simulink model "Electrical_System_2018b_obfs"  (R2019b)
settings: Solver=VariableStepAuto  StartTime=0.0  StopTime=5  RelTol=1e-3  AbsTol=1e-3  EnableMultiTasking=on
InitFcn:
  | Steady_State_Initialisation;
StopFcn:
  | %sscexplore(simlog);
  | %Logging
undefined symbols (not defined in the file): abrlhklxvp, aexgmhuedq, afmfmjnutg, afpphrjpnc, ahuxbyvruc, alarvljztt, amxnyqmnuw, aodrlwvqie, aolhmuplyq, aqpmguuqkg, auesgwirzl, aurophlnng, awamelrhru, ayfhvxflxn, azxkacuhqc, babszerikg, bawhdqanwq, bevoqecvei, bltjvqbchx, bmqsuewujl, bsmyqjfgnf, btvjbsmnve, bywgxqeadw, bziaduxaer, bzmcmdqocb, bzsvyvetat, ccsjnrbsih, cdvenygxwh, cedkrnslhx, cjheorclzs, cjrdshrtqx, ckhavyhcza, ckxewznhlz, cmrcgyiplk, conenicnws, cqkejbgjnn, csfnuwymhe, cunupkhwbh, cwzfvzuxxh, dcadmadufn, dcfponivnv, ddtrqjrhjn, dfhoxvkqas, dfrhtcwpne, dfvomcagjv, djijwylxea, dnmeqksrrm, dnzewbdkaa, dsqcykyxav, dtswwlttmm, ecumpidjtv, edegaywrct, ejjjsmnejc, eknqnehjdz, emvdetzouf, esxbqkbahr, etnkkbreiq, eunoiiiirw, ewewcuedir, fatkfxdhtc ... (+386)
libraries: fl_lib x802, ee_lib x362, fl_ps_legacy_lib x160, nesl_utility x85
(part 24 of 26)

== system Electrical_System_2018b_obfs/Redacted_1221/Redacted_7996/Redacted_9242/Redacted_38/Redacted_8107/Redacted_7529 ==
  Redacted_1084 : ee_lib/Semiconductors & Converters/Diode  ModelType=izdobyzqle  Vf=evihkhstbw V  Ron=vuuzcskhxp Ohm  Goff=mlnvudefzh S  prmExp=lejtfyvyux  I12=tabfzyvjjw A  V12=fmhjbmpmqb V  IS=owmyvxeefr A  ec=svhshwyrgx  I1=ljwwgiysfr A  V1=cxpndjgyrh V  RS=xmnymghsco Ohm  Tmeas=zghhcluqyd degC  N_series=cpqweisfkm  N_parallel=lexvmnvtgk  Rz=qmwaibykde Ohm  BV=drbkvafvno V  C_param=xxddurxsbn  CJ=xdxqdbopkt pF  CJ0=kptwwgjzso pF  VJ=hkmlapdavl V  Mgrad=vyzsmtybaj  Vvec=idvcnbeqxi V  Cvec=lhhotedrtn pF  FC=bewrjixdsy  Q_param=ivgezzsvid  iRM=kttgtaurdl A  iF=feyuhnjntw A  didt=wzaronjtgo A/us  trr_factor=xjeyfathbr  trr=gmgemqpikq ns  Qrr=psqfrowxwi s*uA  TT=klclxejlrf ns  tau=dytmmyuhbl ns  T_param=gahisfowsc  IS_T2=cvrsutiwlp A  I1_T2=lhcryknhzp A  V1_T2=nabkspnaxp V  Tmeas2=yxgzayqlzi degC  EG_param=qwryskkgkm  EG=oxgfzaipim eV  XTI_param=bjoagcqjsw  XTI=ycmlwmcwwf  dBVdT=dotvxllash V/K  Tdevice=ezkzuymnag degC  i_specify=off  i_priority=None  i=daydkonpxs A  i_nominal_specify=off  i_nominal_unit=A  i_nominal_value=blmtdukctw  v_specify=off  v_priority=None  v=akgpvqsdrg V  v_nominal_specify=off  v_nominal_unit=V  v_nominal_value=lygvltjuxz  i_capacitor_specify=off  i_capacitor_priority=None  i_capacitor=btazvuzoqw A  i_capacitor_nominal_specify=off  i_capacitor_nominal_unit=A  i_capacitor_nominal_value=mpfscvienm  v_capacitor_specify=off  v_capacitor_priority=None  v_capacitor=fmmkhztbpm V  v_capacitor_nominal_specify=off  v_capacitor_nominal_unit=V  v_capacitor_nominal_value=ltvznzjvwn  power_dissipated_specify=off  power_dissipated_priority=None  power_dissipated=jxwbertlfp W  power_dissipated_nominal_specify=off  power_dissipated_nominal_unit=W  power_dissipated_nominal_value=qtoemtvmie  thermal_network_parameterization=vtcsjudzim  Rth=heeowetwuv K/W  Rth_Foster=ruqyjqugrl K/W  thermal_mass_parameterization=envbmlquin  thermal_mass=kwknucpqzf J/K  thermal_mass_Foster=cqdqbkuljl J/K  thermal_time_constant=ngzwrugeai s  thermal_time_constant_Foster=bpqkuoqgpu s  thermal_mass_initial_temperatures=rhqgsoeffv degC
      settings: SourceProductName=Simscape Electrical  InternalSimscapePortConfiguration="{\"Bottom\":[],\"Left\":[{\"id\":\"p\",\"label\":\"\",\"type\":\"foundation.electrical.electrical\"},{\"id\":\"H\",\"label\":\"H\",\"type\":\"foundation.thermal.thermal\"}],\"Right\":[{\"id\":\"n\",\"label\":\"\",\"type\":\"foundation.electrical.electrical\"}],\"Top\":[]}"
  Redacted_1116 : ee_lib/Semiconductors & Converters/Diode  ModelType=fezxkqjgqt  Vf=fxigmtorpi V  Ron=gczbijkgdb Ohm  Goff=eezdenrgyt S  prmExp=mooftzwsze  I12=hrjfyjjrls A  V12=rpjtpkqqat V  IS=wddelpkxcd A  ec=wnwrwrhrqv  I1=lxjmeqhfps A  V1=hwunywjuky V  RS=qeymtoopbm Ohm  Tmeas=moiijwwbbr degC  N_series=tpmlovrlqd  N_parallel=mfzinvasat  Rz=ovydxazbex Ohm  BV=pxxjbuwfqz V  C_param=qpcursofjw  CJ=xcjuvsuivt pF  CJ0=izhwoolfnz pF  VJ=vpiestyydi V  Mgrad=cktkfzulrn  Vvec=sciesnzgxa V  Cvec=ffirljqncp pF  FC=ggluskildl  Q_param=ivvyfxrgkf  iRM=vqdtwwvmky A  iF=pvrysfcrbt A  didt=aeuywekxid A/us  trr_factor=nqhyqwmkdj  trr=iqctnvzxva ns  Qrr=isykhlqcxv s*uA  TT=ebdjbikpxl ns  tau=braofdeijp ns  T_param=rwhudzydrl  IS_T2=ahyaxsqykv A  I1_T2=yqxbhliehb A  V1_T2=cahaepnczu V  Tmeas2=rcpxcpgkrc degC  EG_param=ajpcsxcgmn  EG=mkbrzouimp eV  XTI_param=fgrnhizmgq  XTI=rtivxbansn  dBVdT=bztvayfwko V/K  Tdevice=fwkbokttbz degC  i_specify=off  i_priority=None  i=frjerhxssh A  i_nominal_specify=off  i_nominal_unit=A  i_nominal_value=xtkoagasgf  v_specify=off  v_priority=None  v=ltequmallb V  v_nominal_specify=off  v_nominal_unit=V  v_nominal_value=nmmakwdacx  i_capacitor_specify=off  i_capacitor_priority=None  i_capacitor=oexcyamlgf A  i_capacitor_nominal_specify=off  i_capacitor_nominal_unit=A  i_capacitor_nominal_value=tsglkvwluo  v_capacitor_specify=off  v_capacitor_priority=None  v_capacitor=uttypvaate V  v_capacitor_nominal_specify=off  v_capacitor_nominal_unit=V  v_capacitor_nominal_value=rmuymllcxy  power_dissipated_specify=off  power_dissipated_priority=None  power_dissipated=pikztcggua W  power_dissipated_nominal_specify=off  power_dissipated_nominal_unit=W  power_dissipated_nominal_value=wdovbxesnv  thermal_network_parameterization=jzuiubyezr  Rth=zuswrtrzus K/W  Rth_Foster=mncqifigaw K/W  thermal_mass_parameterization=xdyzfyucfr  thermal_mass=digaqnegbt J/K  thermal_mass_Foster=rlibwejjxp J/K  thermal_time_constant=dtpvzfxfdr s  thermal_time_constant_Foster=lltkuepcfr s  thermal_mass_initial_temperatures=qrjsznixcz degC
      settings: SourceProductName=Simscape Electrical  InternalSimscapePortConfiguration="{\"Bottom\":[],\"Left\":[{\"id\":\"p\",\"label\":\"\",\"type\":\"foundation.electrical.electrical\"},{\"id\":\"H\",\"label\":\"H\",\"type\":\"foundation.thermal.thermal\"}],\"Right\":[{\"id\":\"n\",\"label\":\"\",\"type\":\"foundation.electrical.electrical\"}],\"Top\":[]}"
  Redacted_3535 : ee_lib/Passive/Thermal/Thermal Resistor  R=nnovauibfc K/W  T_specify=off  T_priority=None  T=smooypmoft K  T_nominal_specify=off  T_nominal_unit=K  T_nominal_value=kuntnrwjbm  Q_specify=off  Q_priority=None  Q=ffwudhgepl W  Q_nominal_specify=off  Q_nominal_unit=W  Q_nominal_value=dtpumxdoon
      settings: SourceProductName=Simscape Electrical  SourceProductBaseCode=PS  InternalSimscapePortConfiguration="{\"Bottom\":[],\"Left\":[{\"id\":\"A\",\"label\":\"A\",\"type\":\"foundation.thermal.thermal\"}],\"Right\":[{\"id\":\"B\",\"label\":\"B\",\"type\":\"foundation.thermal.thermal\"}],\"Top\":[]}"
  Redacted_4646 : fl_lib/Electrical/Electrical Elements/Switch  R_closed=pqgaemrczs Ohm  G_open=ijstyudrez 1/Ohm  Threshold=xtptocpmir  i_specify=off  i_priority=None  i=ciwbetxiqp A  i_nominal_specify=off  i_nominal_unit=A  i_nominal_value=enaqgcdnlz  v_specify=off  v_priority=None  v=vzxbmtbrih V  v_nominal_specify=off  v_nominal_unit=V  v_nominal_value=wsynujvvrc
      settings: SourceProductName=Simscape
  Redacted_5773 : ee_lib/Passive/Thermal/Thermal Resistor  R=edegaywrct K/W  T_specify=off  T_priority=None  T=ckxewznhlz K  T_nominal_specify=off  T_nominal_unit=K  T_nominal_value=gkohcrexhh  Q_specify=off  Q_priority=None  Q=ubkoftignu W  Q_nominal_specify=off  Q_nominal_unit=W  Q_nominal_value=dmlagltzis
      settings: SourceProductName=Simscape Electrical  SourceProductBaseCode=PS  InternalSimscapePortConfiguration="{\"Bottom\":[],\"Left\":[{\"id\":\"A\",\"label\":\"A\",\"type\":\"foundation.thermal.thermal\"}],\"Right\":[{\"id\":\"B\",\"label\":\"B\",\"type\":\"foundation.thermal.thermal\"}],\"Top\":[]}"
  Redacted_6378 : fl_lib/Electrical/Electrical Elements/Switch  R_closed=whblxebmyo Ohm  G_open=pswlapjyse 1/Ohm  Threshold=pwweavvhgn  i_specify=off  i_priority=None  i=elbzoqtfyk A  i_nominal_specify=off  i_nominal_unit=A  i_nominal_value=sbenumnblt  v_specify=off  v_priority=None  v=vclonruutc V  v_nominal_specify=off  v_nominal_unit=V  v_nominal_value=xzmfluzccj
      settings: SourceProductName=Simscape
  Redacted_6493 : ee_lib/Semiconductors & Converters/Diode  ModelType=vttiaricbl  Vf=ogmshccous V  Ron=clhmvbtmpj Ohm  Goff=qlartobjid S  prmExp=yehkiyfwrf  I12=uxupgfdefd A  V12=fnuyckqxoq V  IS=gijoawrwfl A  ec=jacbxiiccp  I1=fgncvolvfb A  V1=onmmvewocq V  RS=otizmpmqay Ohm  Tmeas=kapmscogpw degC  N_series=qithjwaybs  N_parallel=gzsiinkylg  Rz=mycurxzcbk Ohm  BV=rewmblcdnc V  C_param=whbhsgwygj  CJ=vcfjucyupa pF  CJ0=xlhglqasyv pF  VJ=qosroxbxnj V  Mgrad=hkxiwvlmct  Vvec=oruqsfqddv V  Cvec=sashthzyhc pF  FC=xhlcguewdu  Q_param=ixrezpchhb  iRM=djiqriviqu A  iF=hegkfqrgrh A  didt=xbnqhutjlk A/us  trr_factor=dzlursyiar  trr=ecuaptzqel ns  Qrr=imqebfbhyx s*uA  TT=dymphevecl ns  tau=sblfgxlvjk ns  T_param=xyqfplnupv  IS_T2=uxlhlnzgja A  I1_T2=cyfpvxxmef A  V1_T2=dbwddhswgd V  Tmeas2=zlvkqtpnfx degC  EG_param=fcgsavfugx  EG=jbtqkskxko eV  XTI_param=buvkrschfc  XTI=qctkrmjsmi  dBVdT=kyilrmqoag V/K  Tdevice=tvzbjueohw degC  i_specify=off  i_priority=None  i=wgxzavfjwv A  i_nominal_specify=off  i_nominal_unit=A  i_nominal_value=zeyksugkif  v_specify=off  v_priority=None  v=knzxvrfofm V  v_nominal_specify=off  v_nominal_unit=V  v_nominal_value=chjlmmweiu  i_capacitor_specify=off  i_capacitor_priority=None  i_capacitor=mednscufnd A  i_capacitor_nominal_specify=off  i_capacitor_nominal_unit=A  i_capacitor_nominal_value=leufklsnbm  v_capacitor_specify=off  v_capacitor_priority=None  v_capacitor=xrcvmsmjec V  v_capacitor_nominal_specify=off  v_capacitor_nominal_unit=V  v_capacitor_nominal_value=tbidastozp  power_dissipated_specify=off  power_dissipated_priority=None  power_dissipated=hpegcrwzwe W  power_dissipated_nominal_specify=off  power_dissipated_nominal_unit=W  power_dissipated_nominal_value=ueblnqxpvf  thermal_network_parameterization=hkgyvucefr  Rth=bprjyiudmm K/W  Rth_Foster=bqwxkgbgel K/W  thermal_mass_parameterization=gnzfaualyz  thermal_mass=qgoqgvzmhv J/K  thermal_mass_Foster=lrajjjlskm J/K  thermal_time_constant=ffhhmbgnyr s  thermal_time_constant_Foster=dwjhaccnar s  thermal_mass_initial_temperatures=clzednejpb degC
      settings: SourceProductName=Simscape Electrical  InternalSimscapePortConfiguration="{\"Bottom\":[],\"Left\":[{\"id\":\"p\",\"label\":\"\",\"type\":\"foundation.electrical.electrical\"},{\"id\":\"H\",\"label\":\"H\",\"type\":\"foundation.thermal.thermal\"}],\"Right\":[{\"id\":\"n\",\"label\":\"\",\"type\":\"foundation.electrical.electrical\"}],\"Top\":[]}"
  Redacted_6995 : ee_lib/Semiconductors & Converters/Diode  ModelType=jutammamgf  Vf=phixztrybu V  Ron=wnueokvcjp Ohm  Goff=tlbagzjnli S  prmExp=qepetuupwd  I12=pipfumlpkp A  V12=cvdomcruuy V  IS=caphgfqgul A  ec=bfsyyglqre  I1=chsqwrduxs A  V1=pnvjrtaaxm V  RS=lnonjcbaes Ohm  Tmeas=uqgbdgyiqe degC  N_series=wzcnpegdoc  N_parallel=vzpnmjfana  Rz=jvagvrqcvr Ohm  BV=iowbeuhkbn V  C_param=zuyiiufywv  CJ=iafdabsqml pF  CJ0=krrwskzkzk pF  VJ=hcozynotnd V  Mgrad=qgebppotct  Vvec=rsjrazbslf V  Cvec=tqthplanse pF  FC=ggxesrxcvy  Q_param=npdtukbqqy  iRM=baufngyjqn A  iF=eaqdcbooap A  didt=zpmwgjwvhg A/us  trr_factor=lxzhpepuka  trr=lxionuhlzp ns  Qrr=cedutijpwi s*uA  TT=unwcmeqxzu ns  tau=bqcttgeatr ns  T_param=hnuznnjugk  IS_T2=heqzetlzuz A  I1_T2=zuzqagssvf A  V1_T2=jebzqvibaa V  Tmeas2=liqnbtkzkz degC  EG_param=paovebrsxo  EG=afafawlgir eV  XTI_param=eznhhwiwyq  XTI=pnvwrinkhd  dBVdT=ncvzhuvhdd V/K  Tdevice=xjszywknrp degC  i_specify=off  i_priority=None  i=ksmvescqii A  i_nominal_specify=off  i_nominal_unit=A  i_nominal_value=vdbtoezmns  v_specify=off  v_priority=None  v=mjrlqidlhj V  v_nominal_specify=off  v_nominal_unit=V  v_nominal_value=kpyhvjeelx  i_capacitor_specify=off  i_capacitor_priority=None  i_capacitor=rleowstiyj A  i_capacitor_nominal_specify=off  i_capacitor_nominal_unit=A  i_capacitor_nominal_value=cqjcqxpbep  v_capacitor_specify=off  v_capacitor_priority=None  v_capacitor=atjaslazmh V  v_capacitor_nominal_specify=off  v_capacitor_nominal_unit=V  v_capacitor_nominal_value=wpxewlzklj  power_dissipated_specify=off  power_dissipated_priority=None  power_dissipated=mwdylpnyws W  power_dissipated_nominal_specify=off  power_dissipated_nominal_unit=W  power_dissipated_nominal_value=jrnlbozeni  thermal_network_parameterization=dbphpnpgiy  Rth=xxmcnnlxls K/W  Rth_Foster=owybowsyqi K/W  thermal_mass_parameterization=fipqtfbsom  thermal_mass=sufocoiqer J/K  thermal_mass_Foster=kpdllifdhl J/K  thermal_time_constant=miladgbser s  thermal_time_constant_Foster=ttjplmfpfh s  thermal_mass_initial_temperatures=yzetsrudhm degC
      settings: SourceProductName=Simscape Electrical  InternalSimscapePortConfiguration="{\"Bottom\":[],\"Left\":[{\"id\":\"p\",\"label\":\"\",\"type\":\"foundation.electrical.electrical\"},{\"id\":\"H\",\"label\":\"H\",\"type\":\"foundation.thermal.thermal\"}],\"Right\":[{\"id\":\"n\",\"label\":\"\",\"type\":\"foundation.electrical.electrical\"}],\"Top\":[]}"
  Redacted_7501 : fl_lib/Electrical/Electrical Elements/Switch  R_closed=hkpufaysry Ohm  G_open=gpzouyuqvs 1/Ohm  Threshold=qzaeawbkdg  i_specify=off  i_priority=None  i=gtsknxhqqy A  i_nominal_specify=off  i_nominal_unit=A  i_nominal_value=zlbtgeochj  v_specify=off  v_priority=None  v=dywgqxyfrf V  v_nominal_specify=off  v_nominal_unit=V  v_nominal_value=tmhxabklck
      settings: SourceProductName=Simscape
  Redacted_7912 : ee_lib/Semiconductors & Converters/Diode  ModelType=rwagzwdqyn  Vf=iprlzxekyz V  Ron=ezbutranua Ohm  Goff=dhqmfjsjtj S  prmExp=cuexlqtxbd  I12=huvborskst A  V12=yjowgrbbok V  IS=recqqdaika A  ec=maqoiaeowd  I1=dfgsziufhg A  V1=jfgkxmlxal V  RS=rwxzegglbh Ohm  Tmeas=jioffbrnci degC  N_series=fvxphqozbm  N_parallel=klvniviixg  Rz=lchiewuqih Ohm  BV=jvermwbkfz V  C_param=aeaujmzfqy  CJ=rqoxxznype pF  CJ0=fgmgeudhfq pF  VJ=dirbounqek V  Mgrad=rzoyersdzn  Vvec=uohghsdlzr V  Cvec=sbaqfspfgh pF  FC=nnbelozaaf  Q_param=otgxpunumz  iRM=nvsewfidxu A  iF=stbhkngzcy A  didt=qcdzydoljm A/us  trr_factor=finkzecfng  trr=obgbvrcfxj ns  Qrr=hjehgagare s*uA  TT=fxfsjglodu ns  tau=lgetnnmyzx ns  T_param=mpmzudimoq  IS_T2=ixsjntuwes A  I1_T2=nlkfhnvcta A  V1_T2=ihjdtzpuop V  Tmeas2=tlrwraxkbp degC  EG_param=xxzzjsgowy  EG=osmqxpygwj eV  XTI_param=xnphfrlzyj  XTI=lyfutvjcve  dBVdT=zpjxgnsdoi V/K  Tdevice=ejwhigvruq degC  i_specify=off  i_priority=None  i=fjexkzazrq A  i_nominal_specify=off  i_nominal_unit=A  i_nominal_value=fuktovoelv  v_specify=off  v_priority=None  v=wqxfyskvyj V  v_nominal_specify=off  v_nominal_unit=V  v_nominal_value=kqzybxpjnu  i_capacitor_specify=off  i_capacitor_priority=None  i_capacitor=ofanbrxoer A  i_capacitor_nominal_specify=off  i_capacitor_nominal_unit=A  i_capacitor_nominal_value=joivzqgqdu  v_capacitor_specify=off  v_capacitor_priority=None  v_capacitor=slkzwjrqcn V  v_capacitor_nominal_specify=off  v_capacitor_nominal_unit=V  v_capacitor_nominal_value=btklwtqjaq  power_dissipated_specify=off  power_dissipated_priority=None  power_dissipated=bkyjzqujvp W  power_dissipated_nominal_specify=off  power_dissipated_nominal_unit=W  power_dissipated_nominal_value=wvaevrhbzy  thermal_network_parameterization=ntnnypyupt  Rth=fjtewgrqlr K/W  Rth_Foster=rcjajmoogt K/W  thermal_mass_parameterization=wipcxjewms  thermal_mass=ljwuxclnun J/K  thermal_mass_Foster=llxyimdsaa J/K  thermal_time_constant=dxqpwebpua s  thermal_time_constant_Foster=pglxwtomtd s  thermal_mass_initial_temperatures=hidbrzofoy degC
      settings: SourceProductName=Simscape Electrical  InternalSimscapePortConfiguration="{\"Bottom\":[],\"Left\":[{\"id\":\"p\",\"label\":\"\",\"type\":\"foundation.electrical.electrical\"},{\"id\":\"H\",\"label\":\"H\",\"type\":\"foundation.thermal.thermal\"}],\"Right\":[{\"id\":\"n\",\"label\":\"\",\"type\":\"foundation.electrical.electrical\"}],\"Top\":[]}"
  Redacted_8948 : ee_lib/Semiconductors & Converters/Diode  ModelType=zkbpdzndof  Vf=kzhddisigf V  Ron=dwbhxmmusu Ohm  Goff=bovrirpbke S  prmExp=ivxatfylqk  I12=zvwbuodsjc A  V12=hygnuemoix V  IS=tfwnmkcsyy A  ec=zckyboqwbh  I1=gvubnhdebg A  V1=kunekwhnwv V  RS=ecflormmke Ohm  Tmeas=gtkqfbhchd degC  N_series=zexkrzwhec  N_parallel=wsgrspekur  Rz=shpvzfgjkm Ohm  BV=ccrgfqifiu V  C_param=jqwkikvznj  CJ=pnytyzyvdj pF  CJ0=lnkqhrgppk pF  VJ=uipwhuhyam V  Mgrad=iufkrvrvhb  Vvec=xkhpmfjhdd V  Cvec=uybicdtekz pF  FC=fimwjtluum  Q_param=ctngtcsbuv  iRM=irhzfxednb A  iF=qottmbjvjb A  didt=eltqzqpenk A/us  trr_factor=vqicmosdaw  trr=wqdiphslkd ns  Qrr=xasjjvxkjf s*uA  TT=lfeufmusqp ns  tau=blqvezoiur ns  T_param=okzhatcrhj  IS_T2=cdpladztvs A  I1_T2=cfzfnsrxin A  V1_T2=isvyuxqhap V  Tmeas2=uhkmdahdaa degC  EG_param=hrwywwihcq  EG=euxrsrmpjb eV  XTI_param=yykzdnakfo  XTI=zqzfakywur  dBVdT=yajojhgtsn V/K  Tdevice=hzqpbccwul degC  i_specify=off  i_priority=None  i=nyprrbxiwt A  i_nominal_specify=off  i_nominal_unit=A  i_nominal_value=qchgoadyeu  v_specify=off  v_priority=None  v=cxjaxlbuuh V  v_nominal_specify=off  v_nominal_unit=V  v_nominal_value=enugljpiad  i_capacitor_specify=off  i_capacitor_priority=None  i_capacitor=fyumucjymc A  i_capacitor_nominal_specify=off  i_capacitor_nominal_unit=A  i_capacitor_nominal_value=mwslhozglg  v_capacitor_specify=off  v_capacitor_priority=None  v_capacitor=hatozsragm V  v_capacitor_nominal_specify=off  v_capacitor_nominal_unit=V  v_capacitor_nominal_value=nedivgajsa  power_dissipated_specify=off  power_dissipated_priority=None  power_dissipated=dxpmizpfad W  power_dissipated_nominal_specify=off  power_dissipated_nominal_unit=W  power_dissipated_nominal_value=mfhacyeutq  thermal_network_parameterization=kkiafvbnuz  Rth=dhbknzzzyf K/W  Rth_Foster=krirsjbigm K/W  thermal_mass_parameterization=ncxhbuwddl  thermal_mass=ixwloffvbv J/K  thermal_mass_Foster=ysigxentbo J/K  thermal_time_constant=xcztavzciz s  thermal_time_constant_Foster=ysamghlcvt s  thermal_mass_initial_temperatures=bozfzmyjvc degC
      settings: SourceProductName=Simscape Electrical  InternalSimscapePortConfiguration="{\"Bottom\":[],\"Left\":[{\"id\":\"p\",\"label\":\"\",\"type\":\"foundation.electrical.electrical\"},{\"id\":\"H\",\"label\":\"H\",\"type\":\"foundation.thermal.thermal\"}],\"Right\":[{\"id\":\"n\",\"label\":\"\",\"type\":\"foundation.electrical.electrical\"}],\"Top\":[]}"
  Redacted_9145 : ee_lib/Passive/Thermal/Thermal Resistor  R=ayfhvxflxn K/W  T_specify=off  T_priority=None  T=tjccnrtnkd K  T_nominal_specify=off  T_nominal_unit=K  T_nominal_value=fepcbhdcxp  Q_specify=off  Q_priority=None  Q=yjxepqleci W  Q_nominal_specify=off  Q_nominal_unit=W  Q_nominal_value=ednxibyxiq
      settings: SourceProductName=Simscape Electrical  SourceProductBaseCode=PS  InternalSimscapePortConfiguration="{\"Bottom\":[],\"Left\":[{\"id\":\"A\",\"label\":\"A\",\"type\":\"foundation.thermal.thermal\"}],\"Right\":[{\"id\":\"B\",\"label\":\"B\",\"type\":\"foundation.thermal.thermal\"}],\"Top\":[]}"
  Redacted_9512 : ee_lib/Passive/Thermal/Thermal Resistor  R=qdhdwuufms K/W  T_specify=off  T_priority=None  T=qpsjblfwaq K  T_nominal_specify=off  T_nominal_unit=K  T_nominal_value=jijbdnsmls  Q_specify=off  Q_priority=None  Q=isaanbfiuu W  Q_nominal_specify=off  Q_nominal_unit=W  Q_nominal_value=pquhzcjzlx
      settings: SourceProductName=Simscape Electrical  SourceProductBaseCode=PS  InternalSimscapePortConfiguration="{\"Bottom\":[],\"Left\":[{\"id\":\"A\",\"label\":\"A\",\"type\":\"foundation.thermal.thermal\"}],\"Right\":[{\"id\":\"B\",\"label\":\"B\",\"type\":\"foundation.thermal.thermal\"}],\"Top\":[]}"
  Redacted_3998 : PMIOPort  Side=Left
  Redacted_3025 : PMIOPort  Port=2  Side=Left
  Redacted_376 : PMIOPort  Port=3  Side=Left
  Redacted_4990 : PMIOPort  Port=4  Side=Right
  Redacted_668 : PMIOPort  Port=5  Side=Right
  Redacted_6324 : PMIOPort  Port=6  Side=Right
  Redacted_5539 : PMIOPort  Port=7  Side=Left
  Redacted_7776 : PMIOPort  Port=8  Side=Right
  connections:
  Redacted_9145/LConn1 -- Redacted_1116/LConn2 -- Redacted_6493/LConn2
  Redacted_9512/RConn1 -- Redacted_5539/RConn1
  Redacted_7912/LConn2 -- Redacted_3535/LConn1 -- Redacted_6995/LConn2
  Redacted_7912/RConn1 -- Redacted_7501/LConn1 -- Redacted_6995/LConn1
  Redacted_668/RConn1 -- Redacted_4646/RConn2
  Redacted_6378/RConn1 -- Redacted_4646/RConn1 -- Redacted_7501/RConn1 -- Redacted_7776/RConn1
  Redacted_6324/RConn1 -- Redacted_7501/RConn2
  Redacted_6995/RConn1 -- Redacted_376/RConn1 -- Redacted_7912/LConn1
  Redacted_5773/RConn1 -- Redacted_9512/LConn1 -- Redacted_3535/RConn1 -- Redacted_9145/RConn1
  Redacted_1084/RConn1 -- Redacted_3998/RConn1 -- Redacted_8948/LConn1
  Redacted_8948/RConn1 -- Redacted_6378/LConn1 -- Redacted_1084/LConn1
  Redacted_4990/RConn1 -- Redacted_6378/RConn2
  Redacted_1084/LConn2 -- Redacted_8948/LConn2 -- Redacted_5773/LConn1
  Redacted_1116/LConn1 -- Redacted_4646/LConn1 -- Redacted_6493/RConn1
  Redacted_1116/RConn1 -- Redacted_3025/RConn1 -- Redacted_6493/LConn1

== system Electrical_System_2018b_obfs/Redacted_1221/Redacted_7996/Redacted_9242/Redacted_38/Redacted_8107/Redacted_8444 ==
  Neutral_Negative : Subsystem  VariantControl=Variant1
  Positive_Neutral : Subsystem  VariantControl=Variant3
  Redacted_3917 : Subsystem  VariantControl=Variant2
  Redacted_8974 : PMIOPort  Side=Left
  Redacted_9727 : PMIOPort  Port=2  Side=Left
  Redacted_5818 : PMIOPort  Port=3  Side=Left
  Redacted_9930 : PMIOPort  Port=4  Side=Right
  Redacted_8840 : PMIOPort  Port=5  Side=Right

== system Electrical_System_2018b_obfs/Redacted_1221/Redacted_7996/Redacted_1/Redacted_4377/Redacted_6082/Redacted_144/Neutral_Negative ==
  Open Circuit : fl_lib/Electrical/Electrical Elements/Open Circuit  v_specify=off  v_priority=None  v=0 V  v_nominal_specify=off  v_nominal_unit=V  v_nominal_value=1
      settings: SourceProductName=Simscape  SourceProductBaseCode=SS
  Redacted_3879 : PMIOPort  Side=Left
  Redacted_3368 : PMIOPort  Port=2  Side=Left
  Redacted_9451 : PMIOPort  Port=3  Side=Left
  Redacted_8432 : PMIOPort  Port=4  Side=Right
  Redacted_6806 : PMIOPort  Port=5  Side=Right
  connections:
  Redacted_6806/RConn1 -- Redacted_9451/RConn1
  Open Circuit/LConn1 -- Redacted_3879/RConn1
  Redacted_3368/RConn1 -- Redacted_8432/RConn1

== system Electrical_System_2018b_obfs/Redacted_1221/Redacted_7996/Redacted_1/Redacted_4377/Redacted_6082/Redacted_144/Positive_Neutral ==
  Open Circuit : fl_lib/Electrical/Electrical Elements/Open Circuit  v_specify=off  v_priority=None  v=0 V  v_nominal_specify=off  v_nominal_unit=V  v_nominal_value=1
      settings: SourceProductName=Simscape  SourceProductBaseCode=SS
  Redacted_3879 : PMIOPort  Side=Left
  Redacted_3368 : PMIOPort  Port=2  Side=Left
  Redacted_9451 : PMIOPort  Port=3  Side=Left
  Redacted_8432 : PMIOPort  Port=4  Side=Right
  Redacted_6806 : PMIOPort  Port=5  Side=Right
  connections:
  Open Circuit/LConn1 -- Redacted_9451/RConn1
  Redacted_8432/RConn1 -- Redacted_3879/RConn1
  Redacted_3368/RConn1 -- Redacted_6806/RConn1

== system Electrical_System_2018b_obfs/Redacted_1221/Redacted_7996/Redacted_1/Redacted_4377/Redacted_6082/Redacted_144/Redacted_9503 ==
  Redacted_4565 : fl_lib/Electrical/Electrical Elements/Open Circuit  v_specify=off  v_priority=None  v=skhzijqmdj V  v_nominal_specify=off  v_nominal_unit=V  v_nominal_value=jdqusxliha
      settings: SourceProductName=Simscape  SourceProductBaseCode=SS
  Redacted_3879 : PMIOPort  Side=Left
  Redacted_3368 : PMIOPort  Port=2  Side=Left
  Redacted_9451 : PMIOPort  Port=3  Side=Left
  Redacted_8432 : PMIOPort  Port=4  Side=Right
  Redacted_6806 : PMIOPort  Port=5  Side=Right
  connections:
  Redacted_4565/LConn1 -- Redacted_3368/RConn1
  Redacted_8432/RConn1 -- Redacted_3879/RConn1
  Redacted_6806/RConn1 -- Redacted_9451/RConn1

== system Electrical_System_2018b_obfs/Redacted_1221/Redacted_7996/Redacted_1/Redacted_4377/Redacted_6082/Redacted_1544/Neutral_Negative ==
  Open Circuit : fl_lib/Electrical/Electrical Elements/Open Circuit  v_specify=off  v_priority=None  v=0 V  v_nominal_specify=off  v_nominal_unit=V  v_nominal_value=1
      settings: SourceProductName=Simscape  SourceProductBaseCode=SS
  Redacted_697 : PMIOPort  Side=Left
  Redacted_9789 : PMIOPort  Port=2  Side=Left
  Redacted_5820 : PMIOPort  Port=3  Side=Left
  Redacted_1167 : PMIOPort  Port=4  Side=Right
  Redacted_9408 : PMIOPort  Port=5  Side=Right
  connections:
  Redacted_9408/RConn1 -- Redacted_5820/RConn1
  Open Circuit/LConn1 -- Redacted_697/RConn1
  Redacted_9789/RConn1 -- Redacted_1167/RConn1

== system Electrical_System_2018b_obfs/Redacted_1221/Redacted_7996/Redacted_1/Redacted_4377/Redacted_6082/Redacted_1544/Positive_Neutral ==
  Open Circuit : fl_lib/Electrical/Electrical Elements/Open Circuit  v_specify=off  v_priority=None  v=0 V  v_nominal_specify=off  v_nominal_unit=V  v_nominal_value=1
      settings: SourceProductName=Simscape  SourceProductBaseCode=SS
  Redacted_697 : PMIOPort  Side=Left
  Redacted_9789 : PMIOPort  Port=2  Side=Left
  Redacted_5820 : PMIOPort  Port=3  Side=Left
  Redacted_1167 : PMIOPort  Port=4  Side=Right
  Redacted_9408 : PMIOPort  Port=5  Side=Right
  connections:
  Open Circuit/LConn1 -- Redacted_5820/RConn1
  Redacted_1167/RConn1 -- Redacted_697/RConn1
  Redacted_9789/RConn1 -- Redacted_9408/RConn1

== system Electrical_System_2018b_obfs/Redacted_1221/Redacted_7996/Redacted_1/Redacted_4377/Redacted_6082/Redacted_1544/Redacted_4672 ==
  Redacted_7052 : fl_lib/Electrical/Electrical Elements/Open Circuit  v_specify=off  v_priority=None  v=fpovqwbuex V  v_nominal_specify=off  v_nominal_unit=V  v_nominal_value=qdnyfekgsz
      settings: SourceProductName=Simscape  SourceProductBaseCode=SS
  Redacted_697 : PMIOPort  Side=Left
  Redacted_9789 : PMIOPort  Port=2  Side=Left
  Redacted_5820 : PMIOPort  Port=3  Side=Left
  Redacted_1167 : PMIOPort  Port=4  Side=Right
  Redacted_9408 : PMIOPort  Port=5  Side=Right
  connections:
  Redacted_7052/LConn1 -- Redacted_9789/RConn1
  Redacted_1167/RConn1 -- Redacted_697/RConn1
  Redacted_9408/RConn1 -- Redacted_5820/RConn1

== system Electrical_System_2018b_obfs/Redacted_1221/Redacted_7996/Redacted_1/Redacted_4377/Redacted_6082/Redacted_1843/Neutral_Negative ==
  Open Circuit : fl_lib/Electrical/Electrical Elements/Open Circuit  v_specify=off  v_priority=None  v=0 V  v_nominal_specify=off  v_nominal_unit=V  v_nominal_value=1
      settings: SourceProductName=Simscape  SourceProductBaseCode=SS
  Redacted_2601 : PMIOPort  Side=Left
  Redacted_5367 : PMIOPort  Port=2  Side=Left
  Redacted_1109 : PMIOPort  Port=3  Side=Left
  Redacted_4235 : PMIOPort  Port=4  Side=Right
  Redacted_9086 : PMIOPort  Port=5  Side=Right
  connections:
  Redacted_5367/RConn1 -- Redacted_4235/RConn1
  Open Circuit/LConn1 -- Redacted_2601/RConn1
  Redacted_9086/RConn1 -- Redacted_1109/RConn1

== system Electrical_System_2018b_obfs/Redacted_1221/Redacted_7996/Redacted_1/Redacted_4377/Redacted_6082/Redacted_1843/Positive_Neutral ==
  Open Circuit : fl_lib/Electrical/Electrical Elements/Open Circuit  v_specify=off  v_priority=None  v=0 V  v_nominal_specify=off  v_nominal_unit=V  v_nominal_value=1
      settings: SourceProductName=Simscape  SourceProductBaseCode=SS
  Redacted_2601 : PMIOPort  Side=Left
  Redacted_5367 : PMIOPort  Port=2  Side=Left
  Redacted_1109 : PMIOPort  Port=3  Side=Left
  Redacted_4235 : PMIOPort  Port=4  Side=Right
  Redacted_9086 : PMIOPort  Port=5  Side=Right
  connections:
  Redacted_5367/RConn1 -- Redacted_9086/RConn1
  Redacted_4235/RConn1 -- Redacted_2601/RConn1
  Open Circuit/LConn1 -- Redacted_1109/RConn1

== system Electrical_System_2018b_obfs/Redacted_1221/Redacted_7996/Redacted_1/Redacted_4377/Redacted_6082/Redacted_1843/Redacted_8971 ==
  Redacted_4113 : fl_lib/Electrical/Electrical Elements/Open Circuit  v_specify=off  v_priority=None  v=zogltdvlrz V  v_nominal_specify=off  v_nominal_unit=V  v_nominal_value=pakbffiyvg
      settings: SourceProductName=Simscape  SourceProductBaseCode=SS
  Redacted_2601 : PMIOPort  Side=Left
  Redacted_5367 : PMIOPort  Port=2  Side=Left
  Redacted_1109 : PMIOPort  Port=3  Side=Left
  Redacted_4235 : PMIOPort  Port=4  Side=Right
  Redacted_9086 : PMIOPort  Port=5  Side=Right
  connections:
  Redacted_9086/RConn1 -- Redacted_1109/RConn1
  Redacted_4235/RConn1 -- Redacted_2601/RConn1
  Redacted_4113/LConn1 -- Redacted_5367/RConn1

== system Electrical_System_2018b_obfs/Redacted_1221/Redacted_7996/Redacted_1/Redacted_4377/Redacted_6082/Redacted_2005/Neutral_Negative ==
  Open Circuit : fl_lib/Electrical/Electrical Elements/Open Circuit  v_specify=off  v_priority=None  v=0 V  v_nominal_specify=off  v_nominal_unit=V  v_nominal_value=1
      settings: SourceProductName=Simscape  SourceProductBaseCode=SS
  Redacted_8266 : PMIOPort  Side=Left
  Redacted_1423 : PMIOPort  Port=2  Side=Left
  Redacted_7633 : PMIOPort  Port=3  Side=Left
  Redacted_8552 : PMIOPort  Port=4  Side=Right
  Redacted_2441 : PMIOPort  Port=5  Side=Right
  connections:
  Redacted_1423/RConn1 -- Redacted_8552/RConn1
  Open Circuit/LConn1 -- Redacted_8266/RConn1
  Redacted_2441/RConn1 -- Redacted_7633/RConn1

== system Electrical_System_2018b_obfs/Redacted_1221/Redacted_7996/Redacted_1/Redacted_4377/Redacted_6082/Redacted_2005/Positive_Neutral ==
  Open Circuit : fl_lib/Electrical/Electrical Elements/Open Circuit  v_specify=off  v_priority=None  v=0 V  v_nominal_specify=off  v_nominal_unit=V  v_nominal_value=1
      settings: SourceProductName=Simscape  SourceProductBaseCode=SS
  Redacted_8266 : PMIOPort  Side=Left
  Redacted_1423 : PMIOPort  Port=2  Side=Left
  Redacted_7633 : PMIOPort  Port=3  Side=Left
  Redacted_8552 : PMIOPort  Port=4  Side=Right
  Redacted_2441 : PMIOPort  Port=5  Side=Right
  connections:
  Redacted_1423/RConn1 -- Redacted_2441/RConn1
  Redacted_8552/RConn1 -- Redacted_8266/RConn1
  Open Circuit/LConn1 -- Redacted_7633/RConn1

== system Electrical_System_2018b_obfs/Redacted_1221/Redacted_7996/Redacted_1/Redacted_4377/Redacted_6082/Redacted_2005/Redacted_335 ==
  Redacted_2493 : fl_lib/Electrical/Electrical Elements/Open Circuit  v_specify=off  v_priority=None  v=wmavnefycp V  v_nominal_specify=off  v_nominal_unit=V  v_nominal_value=nysfzchmom
      settings: SourceProductName=Simscape  SourceProductBaseCode=SS
  Redacted_8266 : PMIOPort  Side=Left
  Redacted_1423 : PMIOPort  Port=2  Side=Left
  Redacted_7633 : PMIOPort  Port=3  Side=Left
  Redacted_8552 : PMIOPort  Port=4  Side=Right
  Redacted_2441 : PMIOPort  Port=5  Side=Right
  connections:
  Redacted_2441/RConn1 -- Redacted_7633/RConn1
  Redacted_8552/RConn1 -- Redacted_8266/RConn1
  Redacted_2493/LConn1 -- Redacted_1423/RConn1

== system Electrical_System_2018b_obfs/Redacted_1221/Redacted_7996/Redacted_1/Redacted_4377/Redacted_6082/Redacted_2122/Neutral_Negative ==
  Open Circuit : fl_lib/Electrical/Electrical Elements/Open Circuit  v_specify=off  v_priority=None  v=0 V  v_nominal_specify=off  v_nominal_unit=V  v_nominal_value=1
      settings: SourceProductName=Simscape  SourceProductBaseCode=SS
  Redacted_659 : PMIOPort  Side=Left
  Redacted_1619 : PMIOPort  Port=2  Side=Left
  Redacted_5171 : PMIOPort  Port=3  Side=Left
  Redacted_2219 : PMIOPort  Port=4  Side=Right
  Redacted_5591 : PMIOPort  Port=5  Side=Right
  connections:
  Redacted_1619/RConn1 -- Redacted_2219/RConn1
  Open Circuit/LConn1 -- Redacted_659/RConn1
  Redacted_5591/RConn1 -- Redacted_5171/RConn1

== system Electrical_System_2018b_obfs/Redacted_1221/Redacted_7996/Redacted_1/Redacted_4377/Redacted_6082/Redacted_2122/Positive_Neutral ==
  Open Circuit : fl_lib/Electrical/Electrical Elements/Open Circuit  v_specify=off  v_priority=None  v=0 V  v_nominal_specify=off  v_nominal_unit=V  v_nominal_value=1
      settings: SourceProductName=Simscape  SourceProductBaseCode=SS
  Redacted_659 : PMIOPort  Side=Left
  Redacted_1619 : PMIOPort  Port=2  Side=Left
  Redacted_5171 : PMIOPort  Port=3  Side=Left
  Redacted_2219 : PMIOPort  Port=4  Side=Right
  Redacted_5591 : PMIOPort  Port=5  Side=Right
  connections:
  Redacted_1619/RConn1 -- Redacted_5591/RConn1
  Redacted_2219/RConn1 -- Redacted_659/RConn1
  Open Circuit/LConn1 -- Redacted_5171/RConn1

== system Electrical_System_2018b_obfs/Redacted_1221/Redacted_7996/Redacted_1/Redacted_4377/Redacted_6082/Redacted_2122/Redacted_1391 ==
  Redacted_2352 : fl_lib/Electrical/Electrical Elements/Open Circuit  v_specify=off  v_priority=None  v=jgljlridlh V  v_nominal_specify=off  v_nominal_unit=V  v_nominal_value=owhqxwlzxm
      settings: SourceProductName=Simscape  SourceProductBaseCode=SS
  Redacted_659 : PMIOPort  Side=Left
  Redacted_1619 : PMIOPort  Port=2  Side=Left
  Redacted_5171 : PMIOPort  Port=3  Side=Left
  Redacted_2219 : PMIOPort  Port=4  Side=Right
  Redacted_5591 : PMIOPort  Port=5  Side=Right
  connections:
  Redacted_5591/RConn1 -- Redacted_5171/RConn1
  Redacted_2219/RConn1 -- Redacted_659/RConn1
  Redacted_2352/LConn1 -- Redacted_1619/RConn1

== system Electrical_System_2018b_obfs/Redacted_1221/Redacted_7996/Redacted_1/Redacted_4377/Redacted_6082/Redacted_2443/Neutral_Negative ==
  Open Circuit : fl_lib/Electrical/Electrical Elements/Open Circuit  v_specify=off  v_priority=None  v=0 V  v_nominal_specify=off  v_nominal_unit=V  v_nominal_value=1
      settings: SourceProductName=Simscape  SourceProductBaseCode=SS
  Redacted_2078 : PMIOPort  Side=Left
  Redacted_827 : PMIOPort  Port=2  Side=Left
  Redacted_65 : PMIOPort  Port=3  Side=Left
  Redacted_2555 : PMIOPort  Port=4  Side=Right
  Redacted_7416 : PMIOPort  Port=5  Side=Right
  connections:
  Redacted_827/RConn1 -- Redacted_2555/RConn1
  Open Circuit/LConn1 -- Redacted_2078/RConn1
  Redacted_7416/RConn1 -- Redacted_65/RConn1

== system Electrical_System_2018b_obfs/Redacted_1221/Redacted_7996/Redacted_1/Redacted_4377/Redacted_6082/Redacted_2443/Positive_Neutral ==
  Open Circuit : fl_lib/Electrical/Electrical Elements/Open Circuit  v_specify=off  v_priority=None  v=0 V  v_nominal_specify=off  v_nominal_unit=V  v_nominal_value=1
      settings: SourceProductName=Simscape  SourceProductBaseCode=SS
  Redacted_2078 : PMIOPort  Side=Left
  Redacted_827 : PMIOPort  Port=2  Side=Left
  Redacted_65 : PMIOPort  Port=3  Side=Left
  Redacted_2555 : PMIOPort  Port=4  Side=Right
  Redacted_7416 : PMIOPort  Port=5  Side=Right
  connections:
  Redacted_827/RConn1 -- Redacted_7416/RConn1
  Redacted_2555/RConn1 -- Redacted_2078/RConn1
  Open Circuit/LConn1 -- Redacted_65/RConn1

== system Electrical_System_2018b_obfs/Redacted_1221/Redacted_7996/Redacted_1/Redacted_4377/Redacted_6082/Redacted_2443/Redacted_6791 ==
  Redacted_497 : fl_lib/Electrical/Electrical Elements/Open Circuit  v_specify=off  v_priority=None  v=rijkoulpub V  v_nominal_specify=off  v_nominal_unit=V  v_nominal_value=whtojmaseb
      settings: SourceProductName=Simscape  SourceProductBaseCode=SS
  Redacted_2078 : PMIOPort  Side=Left
  Redacted_827 : PMIOPort  Port=2  Side=Left
  Redacted_65 : PMIOPort  Port=3  Side=Left
  Redacted_2555 : PMIOPort  Port=4  Side=Right
  Redacted_7416 : PMIOPort  Port=5  Side=Right
  connections:
  Redacted_7416/RConn1 -- Redacted_65/RConn1
  Redacted_2555/RConn1 -- Redacted_2078/RConn1
  Redacted_497/LConn1 -- Redacted_827/RConn1

== system Electrical_System_2018b_obfs/Redacted_1221/Redacted_7996/Redacted_1/Redacted_4377/Redacted_6082/Redacted_248/Neutral_Negative ==
  Open Circuit : fl_lib/Electrical/Electrical Elements/Open Circuit  v_specify=off  v_priority=None  v=0 V  v_nominal_specify=off  v_nominal_unit=V  v_nominal_value=1
      settings: SourceProductName=Simscape  SourceProductBaseCode=SS
  Redacted_4518 : PMIOPort  Side=Left
  Redacted_7536 : PMIOPort  Port=2  Side=Left
  Redacted_9561 : PMIOPort  Port=3  Side=Left
  Redacted_1518 : PMIOPort  Port=4  Side=Right
  Redacted_7660 : PMIOPort  Port=5  Side=Right
  connections:
  Redacted_7536/RConn1 -- Redacted_1518/RConn1
  Open Circuit/LConn1 -- Redacted_4518/RConn1
  Redacted_7660/RConn1 -- Redacted_9561/RConn1

== system Electrical_System_2018b_obfs/Redacted_1221/Redacted_7996/Redacted_1/Redacted_4377/Redacted_6082/Redacted_248/Positive_Neutral ==
  Open Circuit : fl_lib/Electrical/Electrical Elements/Open Circuit  v_specify=off  v_priority=None  v=0 V  v_nominal_specify=off  v_nominal_unit=V  v_nominal_value=1
      settings: SourceProductName=Simscape  SourceProductBaseCode=SS
  Redacted_4518 : PMIOPort  Side=Left
  Redacted_7536 : PMIOPort  Port=2  Side=Left
  Redacted_9561 : PMIOPort  Port=3  Side=Left
  Redacted_1518 : PMIOPort  Port=4  Side=Right
  Redacted_7660 : PMIOPort  Port=5  Side=Right
  connections:
  Redacted_7536/RConn1 -- Redacted_7660/RConn1
  Redacted_1518/RConn1 -- Redacted_4518/RConn1
  Open Circuit/LConn1 -- Redacted_9561/RConn1

== system Electrical_System_2018b_obfs/Redacted_1221/Redacted_7996/Redacted_1/Redacted_4377/Redacted_6082/Redacted_248/Redacted_2281 ==
  Redacted_5475 : fl_lib/Electrical/Electrical Elements/Open Circuit  v_specify=off  v_priority=None  v=ayosrghose V  v_nominal_specify=off  v_nominal_unit=V  v_nominal_value=hotsbojhck
      settings: SourceProductName=Simscape  SourceProductBaseCode=SS
  Redacted_4518 : PMIOPort  Side=Left
  Redacted_7536 : PMIOPort  Port=2  Side=Left
  Redacted_9561 : PMIOPort  Port=3  Side=Left
  Redacted_1518 : PMIOPort  Port=4  Side=Right
  Redacted_7660 : PMIOPort  Port=5  Side=Right
  connections:
  Redacted_7660/RConn1 -- Redacted_9561/RConn1
  Redacted_1518/RConn1 -- Redacted_4518/RConn1
  Redacted_5475/LConn1 -- Redacted_7536/RConn1

== system Electrical_System_2018b_obfs/Redacted_1221/Redacted_7996/Redacted_1/Redacted_4377/Redacted_6082/Redacted_2927/Neutral_Negative ==
  Open Circuit : fl_lib/Electrical/Electrical Elements/Open Circuit  v_specify=off  v_priority=None  v=0 V  v_nominal_specify=off  v_nominal_unit=V  v_nominal_value=1
      settings: SourceProductName=Simscape  SourceProductBaseCode=SS
  Redacted_7425 : PMIOPort  Side=Left
  Redacted_110 : PMIOPort  Port=2  Side=Left
  Redacted_9932 : PMIOPort  Port=3  Side=Left
  Redacted_5448 : PMIOPort  Port=4  Side=Right
  Redacted_18 : PMIOPort  Port=5  Side=Right
  connections:
  Redacted_18/RConn1 -- Redacted_9932/RConn1
  Open Circuit/LConn1 -- Redacted_7425/RConn1
  Redacted_110/RConn1 -- Redacted_5448/RConn1

== system Electrical_System_2018b_obfs/Redacted_1221/Redacted_7996/Redacted_1/Redacted_4377/Redacted_6082/Redacted_2927/Positive_Neutral ==
  Open Circuit : fl_lib/Electrical/Electrical Elements/Open Circuit  v_specify=off  v_priority=None  v=0 V  v_nominal_specify=off  v_nominal_unit=V  v_nominal_value=1
      settings: SourceProductName=Simscape  SourceProductBaseCode=SS
  Redacted_7425 : PMIOPort  Side=Left
  Redacted_110 : PMIOPort  Port=2  Side=Left
  Redacted_9932 : PMIOPort  Port=3  Side=Left
  Redacted_5448 : PMIOPort  Port=4  Side=Right
  Redacted_18 : PMIOPort  Port=5  Side=Right
  connections:
  Open Circuit/LConn1 -- Redacted_9932/RConn1
  Redacted_5448/RConn1 -- Redacted_7425/RConn1
  Redacted_110/RConn1 -- Redacted_18/RConn1

== system Electrical_System_2018b_obfs/Redacted_1221/Redacted_7996/Redacted_1/Redacted_4377/Redacted_6082/Redacted_2927/Redacted_9228 ==
  Redacted_5433 : fl_lib/Electrical/Electrical Elements/Open Circuit  v_specify=off  v_priority=None  v=mfngyahdfw V  v_nominal_specify=off  v_nominal_unit=V  v_nominal_value=hwwozmcwbx
      settings: SourceProductName=Simscape  SourceProductBaseCode=SS
  Redacted_7425 : PMIOPort  Side=Left
  Redacted_110 : PMIOPort  Port=2  Side=Left
  Redacted_9932 : PMIOPort  Port=3  Side=Left
  Redacted_5448 : PMIOPort  Port=4  Side=Right
  Redacted_18 : PMIOPort  Port=5  Side=Right
  connections:
  Redacted_5433/LConn1 -- Redacted_110/RConn1
  Redacted_5448/RConn1 -- Redacted_7425/RConn1
  Redacted_18/RConn1 -- Redacted_9932/RConn1

== system Electrical_System_2018b_obfs/Redacted_1221/Redacted_7996/Redacted_1/Redacted_4377/Redacted_6082/Redacted_3086/Neutral_Negative ==
  Open Circuit : fl_lib/Electrical/Electrical Elements/Open Circuit  v_specify=off  v_priority=None  v=0 V  v_nominal_specify=off  v_nominal_unit=V  v_nominal_value=1
      settings: SourceProductName=Simscape  SourceProductBaseCode=SS
  Redacted_6054 : PMIOPort  Side=Left
  Redacted_5626 : PMIOPort  Port=2  Side=Left
  Redacted_6271 : PMIOPort  Port=3  Side=Left
  Redacted_2564 : PMIOPort  Port=4  Side=Right
  Redacted_7933 : PMIOPort  Port=5  Side=Right
  connections:
  Redacted_7933/RConn1 -- Redacted_6271/RConn1
  Open Circuit/LConn1 -- Redacted_6054/RConn1
  Redacted_5626/RConn1 -- Redacted_2564/RConn1

== system Electrical_System_2018b_obfs/Redacted_1221/Redacted_7996/Redacted_1/Redacted_4377/Redacted_6082/Redacted_3086/Positive_Neutral ==
  Open Circuit : fl_lib/Electrical/Electrical Elements/Open Circuit  v_specify=off  v_priority=None  v=0 V  v_nominal_specify=off  v_nominal_unit=V  v_nominal_value=1
      settings: SourceProductName=Simscape  SourceProductBaseCode=SS
  Redacted_6054 : PMIOPort  Side=Left
  Redacted_5626 : PMIOPort  Port=2  Side=Left
  Redacted_6271 : PMIOPort  Port=3  Side=Left
  Redacted_2564 : PMIOPort  Port=4  Side=Right
  Redacted_7933 : PMIOPort  Port=5  Side=Right
  connections:
  Open Circuit/LConn1 -- Redacted_6271/RConn1
  Redacted_2564/RConn1 -- Redacted_6054/RConn1
  Redacted_5626/RConn1 -- Redacted_7933/RConn1

== system Electrical_System_2018b_obfs/Redacted_1221/Redacted_7996/Redacted_1/Redacted_4377/Redacted_6082/Redacted_3086/Redacted_7741 ==
  Redacted_4240 : fl_lib/Electrical/Electrical Elements/Open Circuit  v_specify=off  v_priority=None  v=ebhsjuvrvm V  v_nominal_specify=off  v_nominal_unit=V  v_nominal_value=uogdcjcffr
      settings: SourceProductName=Simscape  SourceProductBaseCode=SS
  Redacted_6054 : PMIOPort  Side=Left
  Redacted_5626 : PMIOPort  Port=2  Side=Left
  Redacted_6271 : PMIOPort  Port=3  Side=Left
  Redacted_2564 : PMIOPort  Port=4  Side=Right
  Redacted_7933 : PMIOPort  Port=5  Side=Right
  connections:
  Redacted_4240/LConn1 -- Redacted_5626/RConn1
  Redacted_2564/RConn1 -- Redacted_6054/RConn1
  Redacted_7933/RConn1 -- Redacted_6271/RConn1

== system Electrical_System_2018b_obfs/Redacted_1221/Redacted_7996/Redacted_1/Redacted_4377/Redacted_6082/Redacted_3818/Neutral_Negative ==
  Open Circuit : fl_lib/Electrical/Electrical Elements/Open Circuit  v_specify=off  v_priority=None  v=0 V  v_nominal_specify=off  v_nominal_unit=V  v_nominal_value=1
      settings: SourceProductName=Simscape  SourceProductBaseCode=SS
  Redacted_558 : PMIOPort  Side=Left
  Redacted_9353 : PMIOPort  Port=2  Side=Left
  Redacted_2763 : PMIOPort  Port=3  Side=Left
  Redacted_5509 : PMIOPort  Port=4  Side=Right
  Redacted_3127 : PMIOPort  Port=5  Side=Right
  connections:
  Redacted_9353/RConn1 -- Redacted_5509/RConn1
  Open Circuit/LConn1 -- Redacted_558/RConn1
  Redacted_3127/RConn1 -- Redacted_2763/RConn1

== system Electrical_System_2018b_obfs/Redacted_1221/Redacted_7996/Redacted_1/Redacted_4377/Redacted_6082/Redacted_3818/Positive_Neutral ==
  Open Circuit : fl_lib/Electrical/Electrical Elements/Open Circuit  v_specify=off  v_priority=None  v=0 V  v_nominal_specify=off  v_nominal_unit=V  v_nominal_value=1
      settings: SourceProductName=Simscape  SourceProductBaseCode=SS
  Redacted_558 : PMIOPort  Side=Left
  Redacted_9353 : PMIOPort  Port=2  Side=Left
  Redacted_2763 : PMIOPort  Port=3  Side=Left
  Redacted_5509 : PMIOPort  Port=4  Side=Right
  Redacted_3127 : PMIOPort  Port=5  Side=Right
  connections:
  Redacted_9353/RConn1 -- Redacted_3127/RConn1
  Redacted_5509/RConn1 -- Redacted_558/RConn1
  Open Circuit/LConn1 -- Redacted_2763/RConn1

== system Electrical_System_2018b_obfs/Redacted_1221/Redacted_7996/Redacted_1/Redacted_4377/Redacted_6082/Redacted_3818/Redacted_7647 ==
  Redacted_9625 : fl_lib/Electrical/Electrical Elements/Open Circuit  v_specify=off  v_priority=None  v=ubfstcorvt V  v_nominal_specify=off  v_nominal_unit=V  v_nominal_value=abvsahtgbf
      settings: SourceProductName=Simscape  SourceProductBaseCode=SS
  Redacted_558 : PMIOPort  Side=Left
  Redacted_9353 : PMIOPort  Port=2  Side=Left
  Redacted_2763 : PMIOPort  Port=3  Side=Left
  Redacted_5509 : PMIOPort  Port=4  Side=Right
  Redacted_3127 : PMIOPort  Port=5  Side=Right
  connections:
  Redacted_3127/RConn1 -- Redacted_2763/RConn1
  Redacted_5509/RConn1 -- Redacted_558/RConn1
  Redacted_9625/LConn1 -- Redacted_9353/RConn1

== system Electrical_System_2018b_obfs/Redacted_1221/Redacted_7996/Redacted_1/Redacted_4377/Redacted_6082/Redacted_4174/Neutral_Negative ==
  Open Circuit : fl_lib/Electrical/Electrical Elements/Open Circuit  v_specify=off  v_priority=None  v=0 V  v_nominal_specify=off  v_nominal_unit=V  v_nominal_value=1
      settings: SourceProductName=Simscape  SourceProductBaseCode=SS
  Redacted_9679 : PMIOPort  Side=Left
  Redacted_9878 : PMIOPort  Port=2  Side=Left
  Redacted_224 : PMIOPort  Port=3  Side=Left
  Redacted_5953 : PMIOPort  Port=4  Side=Right
  Redacted_7639 : PMIOPort  Port=5  Side=Right
  connections:
  Redacted_9878/RConn1 -- Redacted_5953/RConn1
  Open Circuit/LConn1 -- Redacted_9679/RConn1
  Redacted_7639/RConn1 -- Redacted_224/RConn1

== system Electrical_System_2018b_obfs/Redacted_1221/Redacted_7996/Redacted_1/Redacted_4377/Redacted_6082/Redacted_4174/Positive_Neutral ==
  Open Circuit : fl_lib/Electrical/Electrical Elements/Open Circuit  v_specify=off  v_priority=None  v=0 V  v_nominal_specify=off  v_nominal_unit=V  v_nominal_value=1
      settings: SourceProductName=Simscape  SourceProductBaseCode=SS
  Redacted_9679 : PMIOPort  Side=Left
  Redacted_9878 : PMIOPort  Port=2  Side=Left
  Redacted_224 : PMIOPort  Port=3  Side=Left
  Redacted_5953 : PMIOPort  Port=4  Side=Right
  Redacted_7639 : PMIOPort  Port=5  Side=Right
  connections:
  Redacted_9878/RConn1 -- Redacted_7639/RConn1
  Redacted_5953/RConn1 -- Redacted_9679/RConn1
  Open Circuit/LConn1 -- Redacted_224/RConn1

== system Electrical_System_2018b_obfs/Redacted_1221/Redacted_7996/Redacted_1/Redacted_4377/Redacted_6082/Redacted_4174/Redacted_8370 ==
  Redacted_7682 : fl_lib/Electrical/Electrical Elements/Open Circuit  v_specify=off  v_priority=None  v=krmygfnnpy V  v_nominal_specify=off  v_nominal_unit=V  v_nominal_value=lqikwmhyvq
      settings: SourceProductName=Simscape  SourceProductBaseCode=SS
  Redacted_9679 : PMIOPort  Side=Left
  Redacted_9878 : PMIOPort  Port=2  Side=Left
  Redacted_224 : PMIOPort  Port=3  Side=Left
  Redacted_5953 : PMIOPort  Port=4  Side=Right
  Redacted_7639 : PMIOPort  Port=5  Side=Right
  connections:
  Redacted_7639/RConn1 -- Redacted_224/RConn1
  Redacted_5953/RConn1 -- Redacted_9679/RConn1
  Redacted_7682/LConn1 -- Redacted_9878/RConn1

== system Electrical_System_2018b_obfs/Redacted_1221/Redacted_7996/Redacted_1/Redacted_4377/Redacted_6082/Redacted_4278/Neutral_Negative ==
  Open Circuit : fl_lib/Electrical/Electrical Elements/Open Circuit  v_specify=off  v_priority=None  v=0 V  v_nominal_specify=off  v_nominal_unit=V  v_nominal_value=1
      settings: SourceProductName=Simscape  SourceProductBaseCode=SS
  Redacted_1495 : PMIOPort  Side=Left
  Redacted_2064 : PMIOPort  Port=2  Side=Left
  Redacted_9467 : PMIOPort  Port=3  Side=Left
  Redacted_1543 : PMIOPort  Port=4  Side=Right
  Redacted_9491 : PMIOPort  Port=5  Side=Right
  connections:
  Redacted_9491/RConn1 -- Redacted_9467/RConn1
  Open Circuit/LConn1 -- Redacted_1495/RConn1
  Redacted_2064/RConn1 -- Redacted_1543/RConn1

== system Electrical_System_2018b_obfs/Redacted_1221/Redacted_7996/Redacted_1/Redacted_4377/Redacted_6082/Redacted_4278/Positive_Neutral ==
  Open Circuit : fl_lib/Electrical/Electrical Elements/Open Circuit  v_specify=off  v_priority=None  v=0 V  v_nominal_specify=off  v_nominal_unit=V  v_nominal_value=1
      settings: SourceProductName=Simscape  SourceProductBaseCode=SS
  Redacted_1495 : PMIOPort  Side=Left
  Redacted_2064 : PMIOPort  Port=2  Side=Left
  Redacted_9467 : PMIOPort  Port=3  Side=Left
  Redacted_1543 : PMIOPort  Port=4  Side=Right
  Redacted_9491 : PMIOPort  Port=5  Side=Right
  connections:
  Open Circuit/LConn1 -- Redacted_9467/RConn1
  Redacted_1543/RConn1 -- Redacted_1495/RConn1
  Redacted_2064/RConn1 -- Redacted_9491/RConn1

== system Electrical_System_2018b_obfs/Redacted_1221/Redacted_7996/Redacted_1/Redacted_4377/Redacted_6082/Redacted_4278/Redacted_1592 ==
  Redacted_6518 : fl_lib/Electrical/Electrical Elements/Open Circuit  v_specify=off  v_priority=None  v=kniygukgpp V  v_nominal_specify=off  v_nominal_unit=V  v_nominal_value=dzkrotrooy
      settings: SourceProductName=Simscape  SourceProductBaseCode=SS
  Redacted_1495 : PMIOPort  Side=Left
  Redacted_2064 : PMIOPort  Port=2  Side=Left
  Redacted_9467 : PMIOPort  Port=3  Side=Left
  Redacted_1543 : PMIOPort  Port=4  Side=Right
  Redacted_9491 : PMIOPort  Port=5  Side=Right
  connections:
  Redacted_6518/LConn1 -- Redacted_2064/RConn1
  Redacted_1543/RConn1 -- Redacted_1495/RConn1
  Redacted_9491/RConn1 -- Redacted_9467/RConn1

== system Electrical_System_2018b_obfs/Redacted_1221/Redacted_7996/Redacted_1/Redacted_4377/Redacted_6082/Redacted_4413/Neutral_Negative ==
  Open Circuit : fl_lib/Electrical/Electrical Elements/Open Circuit  v_specify=off  v_priority=None  v=0 V  v_nominal_specify=off  v_nominal_unit=V  v_nominal_value=1
      settings: SourceProductName=Simscape  SourceProductBaseCode=SS
  Redacted_9976 : PMIOPort  Side=Left
  Redacted_5180 : PMIOPort  Port=2  Side=Left
  Redacted_6712 : PMIOPort  Port=3  Side=Left
  Redacted_6595 : PMIOPort  Port=4  Side=Right
  Redacted_8408 : PMIOPort  Port=5  Side=Right
  connections:
  Redacted_8408/RConn1 -- Redacted_6712/RConn1
  Open Circuit/LConn1 -- Redacted_9976/RConn1
  Redacted_5180/RConn1 -- Redacted_6595/RConn1
